simulink model "PV_Battery_Model_2"  (R2020a)
settings: Solver=VariableStepAuto  StartTime=0.0  StopTime=10  RelTol=1e-3
undefined symbols (not defined in the file): Acid, Lead
libraries: powerlib x5, dspstat3 x2, re_lib x1, electricdrivelib x1, eePwmGenerator x1, simulink x1
settings Model: Creator=mitch  LastModifiedBy=mitch

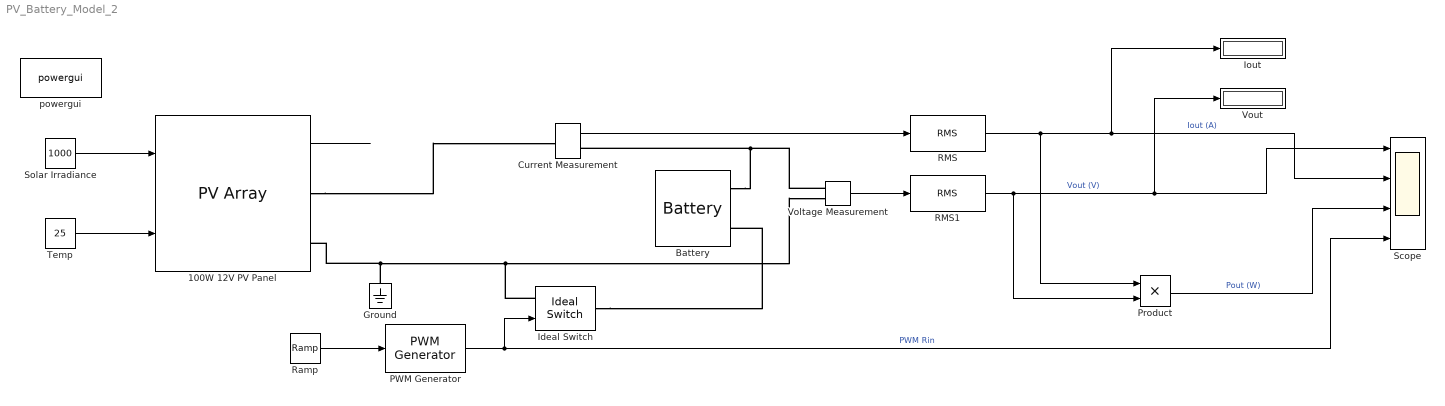
== system PV_Battery_Model_2 ==
  100W 12V PV Panel : re_lib/Solar/PV Array  Npar=1  Nser=1  PlotType=array @ 1000 W/m2 & specified temperatures  S_vec=[ 1000 ]  Temp_C_vec="[ 45 25  ]"  ModuleName=User-defined  PlotWhenSelected=off  Pm=99.9  Ncell=36  Voc=21.6  Isc=6.11  Vm=18  Im=5.55  beta_Voc_pc=-0.38  alpha_Isc_pc=0.05  beta_Voc=-0.08208  alpha_Isc=0.003055  IL=6.1239  I0=3.9408e-10  nI=0.99755  Rsh=64.8707  Rs=0.14729  RobustModel=off  RobustCellTemperature=25  BAL=on  Tc=1e-6  Tfilter=5e-5
  Battery : electricdrivelib/Extra Sources/Battery  BatType=Lead-Acid  ShowTempParam=off  ThermalPreset=no  ShowAgeParam=off  NomV=12  NomQ=7  SOC=80  Batt_Tr=30  PresetModel=on  MaxQ=7.2917  MinV=9  FullV=13.0658  Dis_rate=1.4  R=0.017143  Normal_OP=2.1719  expZone="[12.2171    0.0233333]"  current=[6.5 13 32.5]  Units=Time  Tci=20  NomT=20  T2=-30  MaxQ2=4.8  FullV2=7.1  Normal_OP2=5.655  expZone2="[6.58           1]"  Rca=0.6  ti=2000  Dp=0  Neq0=0  Tsim=1e6  Ta1=25  Qeol=5.4*0.9  Reol=0.013333*1.2  Char_age=[2.3478, 3]  Dis_age=[2.3478, 10]  N1=1500  N2=10500  N3=1000  N4=1400  Ta2=45  N5=950
  Current Measurement : powerlib/Measurements/Current Measurement  PhasorSimulation=off  OutputType=Complex  PSBequivalent=0
  Ground : powerlib/Elements/Ground  LConnTagsString=a
  Ideal Switch : powerlib/Power Electronics/Ideal Switch  Ron=0.001  Lon=0  IC=0  Rs=1e5  Cs=inf  Measurements=off
  Iout : Display
  PWM Generator : eePwmGenerator/PWM Generator  CarrCount=Up  Tper=0.01  Ts=5e-5
  Product : Product
  RMS : dspstat3/RMS  run=on  directionMode=Each column  dimension=1  reset_popup=None
  RMS1 : dspstat3/RMS  run=on  directionMode=Each column  dimension=1  reset_popup=None
  Ramp : simulink/Sources/Ramp  slope=1  start=0  InitialOutput=0
  Scope : Scope  NumInputPorts=4
  Solar Irradiance : Constant  Value=1000
  Temp : Constant  Value=25
  Voltage Measurement : powerlib/Measurements/Voltage Measurement  PhasorSimulation=off  OutputType=Complex  PSBequivalent=0
  Vout : Display
  powergui : powerlib/powergui  Priority=1  SimulationMode=Discrete  SampleTime=5e-05  frequency=60  Iterations=50  frequencyindice=0  Pbase=100e6  ErrMax=1e-4  UnitsV=kV  UnitsW=MW  buscounter=0  FunctionMessages=off  echomessages=off  EnableUseOfTLC=off  CurrentSourceSwitches=off  DisableSnubberDevices=off  DisableRonSwitches=off  DisableVfSwitches=off  DisplayEquations=off  AutomaticDiscreteSolvers=off  SolverType=Tustin/Backward Euler (TBE)  Interpol=off  ExternalGateDelay=off  methode=off  Ts=100  x0status=blocks  SPID=on  SwTol=0  HookPort=off  NonlinearTolerance=1e-4  nMaxIteration=100  ContinueOnMaxIteration=off  RestoreLinks=warning  ResistiveCurrentMeasurement=off  Frange=[0:2:500]  Ylog=off  Xlog=on  ShowGrid=off  save=off  variable=ZData  structure=0  ZoomFFT=off  StartTime=0.0  cycles=1  DisplayStyle=1  fundamental=60  FreqAxis=off  MaxFrequency=1000  frequencyindicesteady=1  RmsSteady=1  display=off
  wires:
  Solar Irradiance/1 -> 100W 12V PV Panel/1
  Ramp/1 -> PWM Generator/1
  PWM Generator/1 -> Ideal Switch/1, Scope/4  "PWM Rin"
  Voltage Measurement/1 -> RMS1/1
  Current Measurement/1 -> RMS/1
  RMS/1 -> Product/1, Iout/1, Scope/2  "Iout (A)"
  RMS1/1 -> Vout/1, Scope/1, Product/2  "Vout (V)"
  Product/1 -> Scope/3  "Pout (W)"
  Temp/1 -> 100W 12V PV Panel/2
  100W 12V PV Panel/1 -> ?
  connections:
  Voltage Measurement/LConn1 -- Battery/LConn1 -- Current Measurement/RConn1
  100W 12V PV Panel/RConn2 -- Ground/LConn1 -- Ideal Switch/LConn1 -- Voltage Measurement/LConn2
  100W 12V PV Panel/RConn1 -- Current Measurement/LConn1
  Ideal Switch/RConn1 -- Battery/LConn2
